simulink model "proj_460_A"  (R2023b)
settings: Solver=VariableStepAuto  StartTime=0.0  StopTime=10  RelTol=1e-3
settings Model: Creator=msa149  LastModifiedBy=msa149

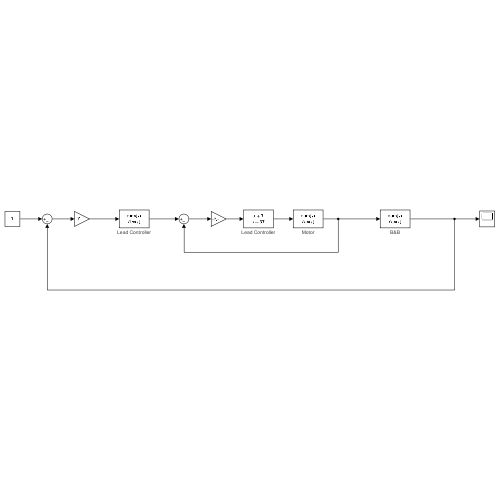
[thumbnail: Simulink's stored preview of the top-level diagram]
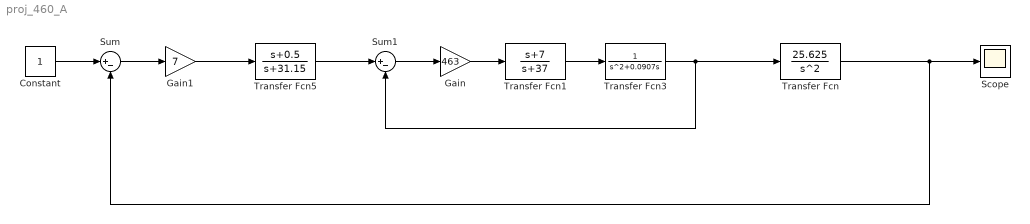
== system proj_460_A ==
  Constant : Constant
  Gain : Gain  Gain=463
  Gain1 : Gain  Gain=7
  Scope : Scope
  Sum : Sum  Inputs=|+-
  Sum1 : Sum  Inputs=|+-
  Transfer Fcn : TransferFcn  Numerator=[25.625]  Denominator=[1 0 0]
      settings: AttributesFormatString=B&B
  Transfer Fcn1 : TransferFcn  Numerator=[1 7]  Denominator=[1 37]
      settings: AttributesFormatString=Lead Controller
  Transfer Fcn3 : TransferFcn  Denominator=[1 0.0907 0]
      settings: AttributesFormatString=Motor
  Transfer Fcn5 : TransferFcn  Numerator=[1 0.5]  Denominator=[1 31.15]
      settings: AttributesFormatString=Lead Controller
  wires:
  Constant/1 -> Sum/1
  Transfer Fcn/1 -> Scope/1, Sum/2
  Transfer Fcn3/1 -> Sum1/2, Transfer Fcn/1
  Transfer Fcn1/1 -> Transfer Fcn3/1
  Sum1/1 -> Gain/1
  Gain/1 -> Transfer Fcn1/1
  Sum/1 -> Gain1/1
  Gain1/1 -> Transfer Fcn5/1
  Transfer Fcn5/1 -> Sum1/1
